simulink library "IO"  (R2024a)
settings: Solver=VariableStepAuto  StartTime=0.0  StopTime=10.0  RelTol=1e-3
values from neighbouring files (symbols this model uses):
  ADCBits = 12.0    [IO.sldd]
  DigitalPolarity : value not decoded    [IO.sldd]
  Vref = 5.0    [IO.sldd]
undefined symbols (not defined in the file or in its folder): Bridge, dt, enum2Raptor, H, raptor_xcp_function
libraries: Raptor_lib x118, Utilities x27, Cooling x1
(part 4 of 4)

== system IO/CANOutputs/Brake ==
  IO_CAN2_151_Bus : Inport
  Bus Selector : BusSelector  OutputSignals=IO_BrakeBias_pct,IO_BrakePressureF_psi,IO_BrakePressureR_psi
  RollingCounterGenerator : Utilities/RollingCounterGenerator
  raptor_can_txmsg : Raptor_lib/CAN/raptor_can_txmsg  canDefinition=struct('dbcFile', 'raptor_CAN2.dbc','message', 'VCU_151','comment', '','signals', {{'VCU_brakeBias','VCU_brakePressureF','VCU_brakePressureR','VCU_counterMsg151'}},'enabled', [ 1 1 1 1;],'scaled', [ 1 1 1 1;],'canBus', '''CAN2''','messageID', [ 151;],'idMask', [ 536870911;],'payloadMask', [],'payloadValue', [],'useDbcPeriod', [ 0;],'period', [ 100;],'queueSize', [ 1;],'label', [ 0;],'ver', [ 2;],'showID', [ 0;],'showRaw', [ 0;],'showRawMsg', [ 0;],'useStartVals', [ 0;],'extendedId', [ 0;],'useSimFunc', [ 0;],'sim_func_name', '''''','fill', [ 0;],'editID', [ 0;],'signalOrder', [ 1;],'signalAscDes', [ 1;],'msgLength', [ 8;])  canBus='CAN2'  queueSize=1  payloadMask=[]  payloadValue=[]  period=100  showID=0  label=0  idMask=hex2dec('1FFFFFFF')  fill=0  id=151  showRaw=0  signalOrder=1  signalInfo={{struct('Name', 'VCU_brakePressureR','StartBit', [ 48;],'SignalSize', [ 16;],'ByteOrder', 'LittleEndian','ValueType', 'SIGNED','Class', 'int16','Signed', [ 1;],'Factor', [ 0.1;],'Offset', [ 0;],'Min', [ 0;],'Max', [ 2000;],'Units', 'psi','StartVal', [ 0;],'Comment', 'Rear brake pressure sensor','Multiplexed', [ 0;],'Multiplexor', [ 0;],'MultiplexMode_Min', [],'MultiplexMode_Max', []),struct('Name', 'VCU_brakePressureF','StartBit', [ 32;],'SignalSize', [ 16;],'ByteOrder', 'LittleEndian','ValueType', 'SIGNED','Class', 'int16','Signed', [ 1;],'Factor', [ 0.1;],'Offset', [ 0;],'Min', [ 0;],'Max', [ 2000;],'Units', 'psi','StartVal', [ 0;],'Comment', 'Front brake pressure sensor','Multiplexed', [ 0;],'Multiplexor', [ 0;],'MultiplexMode_Min', [],'MultiplexMode_Max', []),struct('Name', 'VCU_brakeBias','StartBit', [ 16;],'SignalSize', [ 16;],'ByteOrder', 'LittleEndian','ValueType', 'SIGNED','Class', 'int16','Signed', [ 1;],'Factor', [ 0.1;],'Offset', [ 0;],'Min', [ -3276.8;],'Max', [ 3276.7;],'Units', '%','StartVal', [ 0;],'Comment', 'Brake bias','Multiplexed', [ 0;],'Multiplexor', [ 0;],'MultiplexMode_Min', [],'MultiplexMode_Max', []),struct('Name', 'VCU_counterMsg151','StartBit', [ 0;],'SignalSize', [ 4;],'ByteOrder', 'LittleEndian','ValueType', 'UNSIGNED','Class', 'uint8','Signed', [ 0;],'Factor', [ 1;],'Offset', [ 0;],'Min', [ 0;],'Max', [ 15;],'Units', '','StartVal', [ 0;],'Comment', 'Counter Message 151','Multiplexed', [ 0;],'Multiplexor', [ 0;],'MultiplexMode_Min', [],'MultiplexMode_Max', [])}}  useSimFunc=0  sim_func_name=''  useStartVals=0
      settings: SourceProductName=Raptor
  raptor_function_call_collector : Raptor_lib/Triggers/raptor_function_call_collector  count=10
      settings: SourceProductName=Raptor
  wires:
  raptor_function_call_collector/1 -> RollingCounterGenerator/Trigger
  RollingCounterGenerator/1 -> raptor_can_txmsg/4
  Bus Selector/3 -> raptor_can_txmsg/3  "<IO_BrakePressureR_psi>"
  Bus Selector/1 -> raptor_can_txmsg/1  "<IO_BrakeBias_pct>"
  Bus Selector/2 -> raptor_can_txmsg/2  "<IO_BrakePressureF_psi>"
  IO_CAN2_151_Bus/1 -> Bus Selector/1

== system IO/CANOutputs/DCDC ==
  IO_CAN1_18008FD0_Bus : Inport
  Bus Selector : BusSelector  OutputSignals=IO_DCDCEnable_bool
  Ground : Ground
  raptor_can_txmsg : Raptor_lib/CAN/raptor_can_txmsg  canDefinition=struct('dbcFile', 'raptor_CAN1.dbc','message', 'VCU_18008FD0','comment', '','signals', {{'VCU_dcdcEnable','VCU_dcdcProtect'}},'enabled', [ 1 1;],'scaled', [ 1 1;],'canBus', '''CAN1''','messageID', [ 402690000;],'idMask', [ 536870911;],'payloadMask', [],'payloadValue', [],'useDbcPeriod', [ 0;],'period', [ 100;],'queueSize', [ 1;],'label', [ 0;],'ver', [ 2;],'showID', [ 0;],'showRaw', [ 0;],'showRawMsg', [ 0;],'useStartVals', [ 0;],'extendedId', [ 1;],'useSimFunc', [ 0;],'sim_func_name', '''''','fill', [ 0;],'editID', [ 0;],'signalOrder', [ 1;],'signalAscDes', [ 1;],'msgLength', [ 8;])  canBus='CAN1'  queueSize=1  payloadMask=[]  payloadValue=[]  period=100  showID=0  label=0  idMask=hex2dec('1FFFFFFF')  fill=0  id=402690000  showRaw=0  signalOrder=1  signalInfo={{struct('Name', 'VCU_dcdcProtect','StartBit', [ 2;],'SignalSize', [ 2;],'ByteOrder', 'BigEndian','ValueType', 'UNSIGNED','Class', 'uint8','Signed', [ 0;],'Factor', [ 1;],'Offset', [ 0;],'Min', [ 0;],'Max', [ 0;],'Units', '','StartVal', [ 0;],'Comment', 'Protect command - once commanded, converter won`t work until restart (decimal); 1: protection confirmed','Multiplexed', [ 0;],'Multiplexor', [ 0;],'MultiplexMode_Min', [],'MultiplexMode_Max', []),struct('Name', 'VCU_dcdcEnable','StartBit', [ 0;],'SignalSize', [ 2;],'ByteOrder', 'BigEndian','ValueType', 'UNSIGNED','Class', 'uint8','Signed', [ 0;],'Factor', [ 1;],'Offset', [ 0;],'Min', [ 0;],'Max', [ 0;],'Units', '','StartVal', [ 0;],'Comment', 'Enable command (decimal); 1: enable, 2: disable','Multiplexed', [ 0;],'Multiplexor', [ 0;],'MultiplexMode_Min', [],'MultiplexMode_Max', [])}}  useSimFunc=0  sim_func_name=''  useStartVals=0
      settings: SourceProductName=Raptor
  wires:
  Ground/1 -> raptor_can_txmsg/2
  Bus Selector/1 -> raptor_can_txmsg/1  "<IO_DCDCEnable_bool>"
  IO_CAN1_18008FD0_Bus/1 -> Bus Selector/1

== system IO/CANOutputs/Front Left Tire Temp ==
  IO_CAN2_156_Bus : Inport
  Bus Selector : BusSelector  OutputSignals=IN_TireTempFLI_degC,IN_TireTempFLM_degC,IN_TireTempFLO_degC
  RollingCounterGenerator : Utilities/RollingCounterGenerator
  raptor_can_txmsg : Raptor_lib/CAN/raptor_can_txmsg  canDefinition=struct('dbcFile', 'raptor_CAN2.dbc','message', 'VCU_156','comment', '','signals', {{'VCU_counterMsg156','VCU_tireTempFLI','VCU_tireTempFLM','VCU_tireTempFLO'}},'enabled', [ 1 1 1 1;],'scaled', [ 1 1 1 1;],'canBus', '''CAN2''','messageID', [ 156;],'idMask', [ 536870911;],'payloadMask', [],'payloadValue', [],'useDbcPeriod', [ 0;],'period', [ 100;],'queueSize', [ 1;],'label', [ 0;],'ver', [ 2;],'showID', [ 0;],'showRaw', [ 0;],'showRawMsg', [ 0;],'useStartVals', [ 0;],'extendedId', [ 0;],'useSimFunc', [ 0;],'sim_func_name', '''''','fill', [ 0;],'editID', [ 0;],'signalOrder', [ 1;],'signalAscDes', [ 1;],'msgLength', [ 8;])  canBus='CAN2'  queueSize=1  payloadMask=[]  payloadValue=[]  period=100  showID=0  label=0  idMask=hex2dec('1FFFFFFF')  fill=0  id=156  showRaw=0  signalOrder=1  signalInfo={{struct('Name', 'VCU_counterMsg156','StartBit', [ 0;],'SignalSize', [ 4;],'ByteOrder', 'LittleEndian','ValueType', 'UNSIGNED','Class', 'uint8','Signed', [ 0;],'Factor', [ 1;],'Offset', [ 0;],'Min', [ 0;],'Max', [ 15;],'Units', '','StartVal', [ 0;],'Comment', 'Counter Message 156','Multiplexed', [ 0;],'Multiplexor', [ 0;],'MultiplexMode_Min', [],'MultiplexMode_Max', []),struct('Name', 'VCU_tireTempFLI','StartBit', [ 16;],'SignalSize', [ 16;],'ByteOrder', 'LittleEndian','ValueType', 'SIGNED','Class', 'int16','Signed', [ 1;],'Factor', [ 0.1;],'Offset', [ 0;],'Min', [ -3276.8;],'Max', [ 3276.7;],'Units', 'degC','StartVal', [ 0;],'Comment', 'FLI tire temperature','Multiplexed', [ 0;],'Multiplexor', [ 0;],'MultiplexMode_Min', [],'MultiplexMode_Max', []),struct('Name', 'VCU_tireTempFLM','StartBit', [ 32;],'SignalSize', [ 16;],'ByteOrder', 'LittleEndian','ValueType', 'SIGNED','Class', 'int16','Signed', [ 1;],'Factor', [ 0.1;],'Offset', [ 0;],'Min', [ -3276.8;],'Max', [ 3276.7;],'Units', 'degC','StartVal', [ 0;],'Comment', 'FLM tire temperature','Multiplexed', [ 0;],'Multiplexor', [ 0;],'MultiplexMode_Min', [],'MultiplexMode_Max', []),struct('Name', 'VCU_tireTempFLO','StartBit', [ 48;],'SignalSize', [ 16;],'ByteOrder', 'LittleEndian','ValueType', 'SIGNED','Class', 'int16','Signed', [ 1;],'Factor', [ 0.1;],'Offset', [ 0;],'Min', [ -3276.8;],'Max', [ 3276.7;],'Units', 'degC','StartVal', [ 0;],'Comment', 'FLO tire temperature','Multiplexed', [ 0;],'Multiplexor', [ 0;],'MultiplexMode_Min', [],'MultiplexMode_Max', [])}}  useSimFunc=0  sim_func_name=''  useStartVals=0
      settings: SourceProductName=Raptor
  raptor_function_call_collector : Raptor_lib/Triggers/raptor_function_call_collector  count=10
      settings: SourceProductName=Raptor
  wires:
  raptor_function_call_collector/1 -> RollingCounterGenerator/Trigger
  RollingCounterGenerator/1 -> raptor_can_txmsg/1
  Bus Selector/3 -> raptor_can_txmsg/4  "<IN_TireTempFLO_degC>"
  Bus Selector/2 -> raptor_can_txmsg/3  "<IN_TireTempFLM_degC>"
  Bus Selector/1 -> raptor_can_txmsg/2  "<IN_TireTempFLI_degC>"
  IO_CAN2_156_Bus/1 -> Bus Selector/1

== system IO/CANOutputs/Front Right Tire Temp ==
  IO_CAN2_157_Bus : Inport
  Bus Selector : BusSelector  OutputSignals=IN_TireTempFRI_degC,IN_TireTempFRM_degC,IN_TireTempFRO_degC
  RollingCounterGenerator : Utilities/RollingCounterGenerator
  raptor_can_txmsg : Raptor_lib/CAN/raptor_can_txmsg  canDefinition=struct('dbcFile', 'raptor_CAN2.dbc','message', 'VCU_157','comment', '','signals', {{'VCU_counterMsg157','VCU_tireTempFRI','VCU_tireTempFRM','VCU_tireTempFRO'}},'enabled', [ 1 1 1 1;],'scaled', [ 1 1 1 1;],'canBus', '''CAN2''','messageID', [ 157;],'idMask', [ 536870911;],'payloadMask', [],'payloadValue', [],'useDbcPeriod', [ 0;],'period', [ 100;],'queueSize', [ 1;],'label', [ 0;],'ver', [ 2;],'showID', [ 0;],'showRaw', [ 0;],'showRawMsg', [ 0;],'useStartVals', [ 0;],'extendedId', [ 0;],'useSimFunc', [ 0;],'sim_func_name', '''''','fill', [ 0;],'editID', [ 0;],'signalOrder', [ 1;],'signalAscDes', [ 1;],'msgLength', [ 8;])  canBus='CAN2'  queueSize=1  payloadMask=[]  payloadValue=[]  period=100  showID=0  label=0  idMask=hex2dec('1FFFFFFF')  fill=0  id=157  showRaw=0  signalOrder=1  signalInfo={{struct('Name', 'VCU_counterMsg157','StartBit', [ 0;],'SignalSize', [ 4;],'ByteOrder', 'LittleEndian','ValueType', 'UNSIGNED','Class', 'uint8','Signed', [ 0;],'Factor', [ 1;],'Offset', [ 0;],'Min', [ 0;],'Max', [ 15;],'Units', '','StartVal', [ 0;],'Comment', 'Counter Message 157','Multiplexed', [ 0;],'Multiplexor', [ 0;],'MultiplexMode_Min', [],'MultiplexMode_Max', []),struct('Name', 'VCU_tireTempFRI','StartBit', [ 16;],'SignalSize', [ 16;],'ByteOrder', 'LittleEndian','ValueType', 'SIGNED','Class', 'int16','Signed', [ 1;],'Factor', [ 0.1;],'Offset', [ 0;],'Min', [ -3276.8;],'Max', [ 3276.7;],'Units', 'degC','StartVal', [ 0;],'Comment', 'FRI tire temperature','Multiplexed', [ 0;],'Multiplexor', [ 0;],'MultiplexMode_Min', [],'MultiplexMode_Max', []),struct('Name', 'VCU_tireTempFRM','StartBit', [ 32;],'SignalSize', [ 16;],'ByteOrder', 'LittleEndian','ValueType', 'SIGNED','Class', 'int16','Signed', [ 1;],'Factor', [ 0.1;],'Offset', [ 0;],'Min', [ -3276.8;],'Max', [ 3276.7;],'Units', 'degC','StartVal', [ 0;],'Comment', 'FRM tire temperature','Multiplexed', [ 0;],'Multiplexor', [ 0;],'MultiplexMode_Min', [],'MultiplexMode_Max', []),struct('Name', 'VCU_tireTempFRO','StartBit', [ 48;],'SignalSize', [ 16;],'ByteOrder', 'LittleEndian','ValueType', 'SIGNED','Class', 'int16','Signed', [ 1;],'Factor', [ 0.1;],'Offset', [ 0;],'Min', [ -3276.8;],'Max', [ 3276.7;],'Units', 'degC','StartVal', [ 0;],'Comment', 'FRO tire temperature','Multiplexed', [ 0;],'Multiplexor', [ 0;],'MultiplexMode_Min', [],'MultiplexMode_Max', [])}}  useSimFunc=0  sim_func_name=''  useStartVals=0
      settings: SourceProductName=Raptor
  raptor_function_call_collector : Raptor_lib/Triggers/raptor_function_call_collector  count=10
      settings: SourceProductName=Raptor
  wires:
  raptor_function_call_collector/1 -> RollingCounterGenerator/Trigger
  RollingCounterGenerator/1 -> raptor_can_txmsg/1
  Bus Selector/3 -> raptor_can_txmsg/4  "<IN_TireTempFRO_degC>"
  Bus Selector/2 -> raptor_can_txmsg/3  "<IN_TireTempFRM_degC>"
  Bus Selector/1 -> raptor_can_txmsg/2  "<IN_TireTempFRI_degC>"
  IO_CAN2_157_Bus/1 -> Bus Selector/1

== system IO/CANOutputs/Front Rotor Temp ==
  IO_CAN2_154_Bus : Inport
  Bus Selector : BusSelector  OutputSignals=IN_RotorTempFL_degC,IN_RotorTempFR_degC
  RollingCounterGenerator : Utilities/RollingCounterGenerator
  raptor_can_txmsg : Raptor_lib/CAN/raptor_can_txmsg  canDefinition=struct('dbcFile', 'raptor_CAN2.dbc','message', 'VCU_154','comment', '','signals', {{'VCU_counterMsg154','VCU_rotorTempFL','VCU_rotorTempFR'}},'enabled', [ 1 1 1;],'scaled', [ 1 1 1;],'canBus', '''CAN2''','messageID', [ 154;],'idMask', [ 536870911;],'payloadMask', [],'payloadValue', [],'useDbcPeriod', [ 0;],'period', [ 100;],'queueSize', [ 1;],'label', [ 0;],'ver', [ 2;],'showID', [ 0;],'showRaw', [ 0;],'showRawMsg', [ 0;],'useStartVals', [ 0;],'extendedId', [ 0;],'useSimFunc', [ 0;],'sim_func_name', '''''','fill', [ 0;],'editID', [ 0;],'signalOrder', [ 1;],'signalAscDes', [ 1;],'msgLength', [ 8;])  canBus='CAN2'  queueSize=1  payloadMask=[]  payloadValue=[]  period=100  showID=0  label=0  idMask=hex2dec('1FFFFFFF')  fill=0  id=154  showRaw=0  signalOrder=1  signalInfo={{struct('Name', 'VCU_counterMsg154','StartBit', [ 0;],'SignalSize', [ 4;],'ByteOrder', 'LittleEndian','ValueType', 'UNSIGNED','Class', 'uint8','Signed', [ 0;],'Factor', [ 1;],'Offset', [ 0;],'Min', [ 0;],'Max', [ 15;],'Units', '','StartVal', [ 0;],'Comment', 'Counter Message 154','Multiplexed', [ 0;],'Multiplexor', [ 0;],'MultiplexMode_Min', [],'MultiplexMode_Max', []),struct('Name', 'VCU_rotorTempFL','StartBit', [ 16;],'SignalSize', [ 16;],'ByteOrder', 'LittleEndian','ValueType', 'SIGNED','Class', 'int16','Signed', [ 1;],'Factor', [ 0.1;],'Offset', [ 0;],'Min', [ -3276.8;],'Max', [ 3276.7;],'Units', 'degC','StartVal', [ 0;],'Comment', 'FL rotor temperature','Multiplexed', [ 0;],'Multiplexor', [ 0;],'MultiplexMode_Min', [],'MultiplexMode_Max', []),struct('Name', 'VCU_rotorTempFR','StartBit', [ 32;],'SignalSize', [ 16;],'ByteOrder', 'LittleEndian','ValueType', 'SIGNED','Class', 'int16','Signed', [ 1;],'Factor', [ 0.1;],'Offset', [ 0;],'Min', [ -3276.8;],'Max', [ 3276.7;],'Units', 'degC','StartVal', [ 0;],'Comment', '','Multiplexed', [ 0;],'Multiplexor', [ 0;],'MultiplexMode_Min', [],'MultiplexMode_Max', [])}}  useSimFunc=0  sim_func_name=''  useStartVals=0
      settings: SourceProductName=Raptor
  raptor_function_call_collector : Raptor_lib/Triggers/raptor_function_call_collector  count=10
      settings: SourceProductName=Raptor
  wires:
  RollingCounterGenerator/1 -> raptor_can_txmsg/1
  raptor_function_call_collector/1 -> RollingCounterGenerator/Trigger
  Bus Selector/2 -> raptor_can_txmsg/3  "<IN_RotorTempFR_degC>"
  Bus Selector/1 -> raptor_can_txmsg/2  "<IN_RotorTempFL_degC>"
  IO_CAN2_154_Bus/1 -> Bus Selector/1

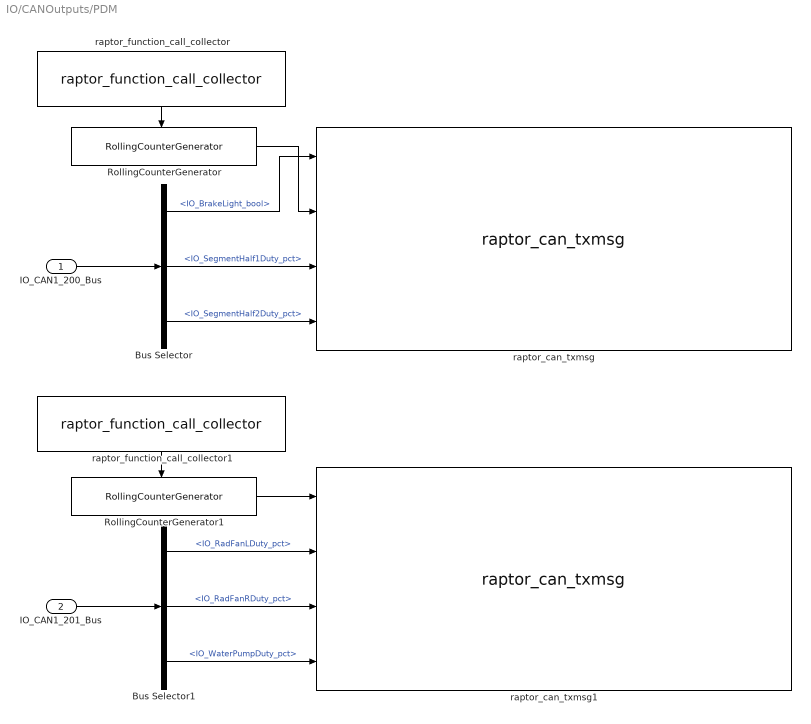
== system IO/CANOutputs/PDM ==
  IO_CAN1_200_Bus : Inport
  IO_CAN1_201_Bus : Inport  Port=2
  Bus Selector : BusSelector  OutputSignals=IO_BrakeLight_bool,IO_SegmentHalf1Duty_pct,IO_SegmentHalf2Duty_pct
  Bus Selector1 : BusSelector  OutputSignals=IO_RadFanLDuty_pct,IO_RadFanRDuty_pct,IO_WaterPumpDuty_pct
  RollingCounterGenerator : Utilities/RollingCounterGenerator
  RollingCounterGenerator1 : Utilities/RollingCounterGenerator
  raptor_can_txmsg : Raptor_lib/CAN/raptor_can_txmsg  canDefinition=struct('dbcFile', 'raptor_CAN1.dbc','message', 'VCU_200','comment', '','signals', {{'VCU_brakeLightCmd','VCU_counterMsg200','VCU_segmentHalf1Duty','VCU_segmentHalf2Duty'}},'enabled', [ 1 1 1 1;],'scaled', [ 1 1 1 1;],'canBus', '''CAN1''','messageID', [ 200;],'idMask', [ 536870911;],'payloadMask', [],'payloadValue', [],'useDbcPeriod', [ 0;],'period', [ 100;],'queueSize', [ 1;],'label', [ 0;],'ver', [ 2;],'showID', [ 0;],'showRaw', [ 0;],'showRawMsg', [ 0;],'useStartVals', [ 0;],'extendedId', [ 0;],'useSimFunc', [ 0;],'sim_func_name', '''''','fill', [ 0;],'editID', [ 0;],'signalOrder', [ 1;],'signalAscDes', [ 1;],'msgLength', [ 8;])  canBus='CAN1'  queueSize=1  payloadMask=[]  payloadValue=[]  period=100  showID=0  label=0  idMask=hex2dec('1FFFFFFF')  fill=0  id=200  showRaw=0  signalOrder=1  signalInfo={{struct('Name', 'VCU_segmentHalf2Duty','StartBit', [ 32;],'SignalSize', [ 16;],'ByteOrder', 'LittleEndian','ValueType', 'SIGNED','Class', 'int16','Signed', [ 1;],'Factor', [ 0.1;],'Offset', [ 0;],'Min', [ 0;],'Max', [ 100;],'Units', '%','StartVal', [ 0;],'Comment', 'Segment half 2 duty','Multiplexed', [ 0;],'Multiplexor', [ 0;],'MultiplexMode_Min', [],'MultiplexMode_Max', []),struct('Name', 'VCU_segmentHalf1Duty','StartBit', [ 16;],'SignalSize', [ 16;],'ByteOrder', 'LittleEndian','ValueType', 'SIGNED','Class', 'int16','Signed', [ 1;],'Factor', [ 0.1;],'Offset', [ 0;],'Min', [ 0;],'Max', [ 100;],'Units', '%','StartVal', [ 0;],'Comment', 'Segment half 1 duty','Multiplexed', [ 0;],'Multiplexor', [ 0;],'MultiplexMode_Min', [],'MultiplexMode_Max', []),struct('Name', 'VCU_brakeLightCmd','StartBit', [ 8;],'SignalSize', [ 1;],'ByteOrder', 'LittleEndian','ValueType', 'UNSIGNED','Class', 'uint8','Signed', [ 0;],'Factor', [ 1;],'Offset', [ 0;],'Min', [ 0;],'Max', [ 1;],'Units', '','StartVal', [ 0;],'Comment', 'Brake light command','Multiplexed', [ 0;],'Multiplexor', [ 0;],'MultiplexMode_Min', [],'MultiplexMode_Max', []),struct('Name', 'VCU_counterMsg200','StartBit', [ 0;],'SignalSize', [ 4;],'ByteOrder', 'LittleEndian','ValueType', 'UNSIGNED','Class', 'uint8','Signed', [ 0;],'Factor', [ 1;],'Offset', [ 0;],'Min', [ 0;],'Max', [ 15;],'Units', '','StartVal', [ 0;],'Comment', 'Counter Message 200','Multiplexed', [ 0;],'Multiplexor', [ 0;],'MultiplexMode_Min', [],'MultiplexMode_Max', [])}}  useSimFunc=0  sim_func_name=''  useStartVals=0
      settings: SourceProductName=Raptor
  raptor_can_txmsg1 : Raptor_lib/CAN/raptor_can_txmsg  canDefinition=struct('dbcFile', 'raptor_CAN1.dbc','message', 'VCU_201','comment', '','signals', {{'VCU_counterMsg201','VCU_radFanLDuty','VCU_radFanRDuty','VCU_waterPumpDuty'}},'enabled', [ 1 1 1 1;],'scaled', [ 1 1 1 1;],'canBus', '''CAN1''','messageID', [ 201;],'idMask', [ 536870911;],'payloadMask', [],'payloadValue', [],'useDbcPeriod', [ 0;],'period', [ 100;],'queueSize', [ 1;],'label', [ 0;],'ver', [ 2;],'showID', [ 0;],'showRaw', [ 0;],'showRawMsg', [ 0;],'useStartVals', [ 0;],'extendedId', [ 0;],'useSimFunc', [ 0;],'sim_func_name', '''''','fill', [ 0;],'editID', [ 0;],'signalOrder', [ 1;],'signalAscDes', [ 1;],'msgLength', [ 8;])  canBus='CAN1'  queueSize=1  payloadMask=[]  payloadValue=[]  period=100  showID=0  label=0  idMask=hex2dec('1FFFFFFF')  fill=0  id=201  showRaw=0  signalOrder=1  signalInfo={{struct('Name', 'VCU_waterPumpDuty','StartBit', [ 48;],'SignalSize', [ 16;],'ByteOrder', 'LittleEndian','ValueType', 'SIGNED','Class', 'int16','Signed', [ 1;],'Factor', [ 0.1;],'Offset', [ 0;],'Min', [ 0;],'Max', [ 100;],'Units', '%','StartVal', [ 0;],'Comment', 'Water pump duty','Multiplexed', [ 0;],'Multiplexor', [ 0;],'MultiplexMode_Min', [],'MultiplexMode_Max', []),struct('Name', 'VCU_radFanRDuty','StartBit', [ 32;],'SignalSize', [ 16;],'ByteOrder', 'LittleEndian','ValueType', 'SIGNED','Class', 'int16','Signed', [ 1;],'Factor', [ 0.1;],'Offset', [ 0;],'Min', [ 0;],'Max', [ 100;],'Units', '%','StartVal', [ 0;],'Comment', 'Right radiator fan duty','Multiplexed', [ 0;],'Multiplexor', [ 0;],'MultiplexMode_Min', [],'MultiplexMode_Max', []),struct('Name', 'VCU_radFanLDuty','StartBit', [ 16;],'SignalSize', [ 16;],'ByteOrder', 'LittleEndian','ValueType', 'SIGNED','Class', 'int16','Signed', [ 1;],'Factor', [ 0.1;],'Offset', [ 0;],'Min', [ 0;],'Max', [ 100;],'Units', '%','StartVal', [ 0;],'Comment', 'Left radiator fan duty','Multiplexed', [ 0;],'Multiplexor', [ 0;],'MultiplexMode_Min', [],'MultiplexMode_Max', []),struct('Name', 'VCU_counterMsg201','StartBit', [ 0;],'SignalSize', [ 4;],'ByteOrder', 'LittleEndian','ValueType', 'UNSIGNED','Class', 'uint8','Signed', [ 0;],'Factor', [ 1;],'Offset', [ 0;],'Min', [ 0;],'Max', [ 15;],'Units', '','StartVal', [ 0;],'Comment', 'Counter Message 201','Multiplexed', [ 0;],'Multiplexor', [ 0;],'MultiplexMode_Min', [],'MultiplexMode_Max', [])}}  useSimFunc=0  sim_func_name=''  useStartVals=0
      settings: SourceProductName=Raptor
  raptor_function_call_collector : Raptor_lib/Triggers/raptor_function_call_collector  count=10
      settings: SourceProductName=Raptor
  raptor_function_call_collector1 : Raptor_lib/Triggers/raptor_function_call_collector  count=10
      settings: SourceProductName=Raptor
  wires:
  raptor_function_call_collector1/1 -> RollingCounterGenerator1/Trigger
  RollingCounterGenerator1/1 -> raptor_can_txmsg1/1
  Bus Selector1/1 -> raptor_can_txmsg1/2  "<IO_RadFanLDuty_pct>"
  Bus Selector1/3 -> raptor_can_txmsg1/4  "<IO_WaterPumpDuty_pct>"
  Bus Selector1/2 -> raptor_can_txmsg1/3  "<IO_RadFanRDuty_pct>"
  IO_CAN1_201_Bus/1 -> Bus Selector1/1
  raptor_function_call_collector/1 -> RollingCounterGenerator/Trigger
  RollingCounterGenerator/1 -> raptor_can_txmsg/2
  Bus Selector/1 -> raptor_can_txmsg/1  "<IO_BrakeLight_bool>"
  Bus Selector/3 -> raptor_can_txmsg/4  "<IO_SegmentHalf2Duty_pct>"
  Bus Selector/2 -> raptor_can_txmsg/3  "<IO_SegmentHalf1Duty_pct>"
  IO_CAN1_200_Bus/1 -> Bus Selector/1

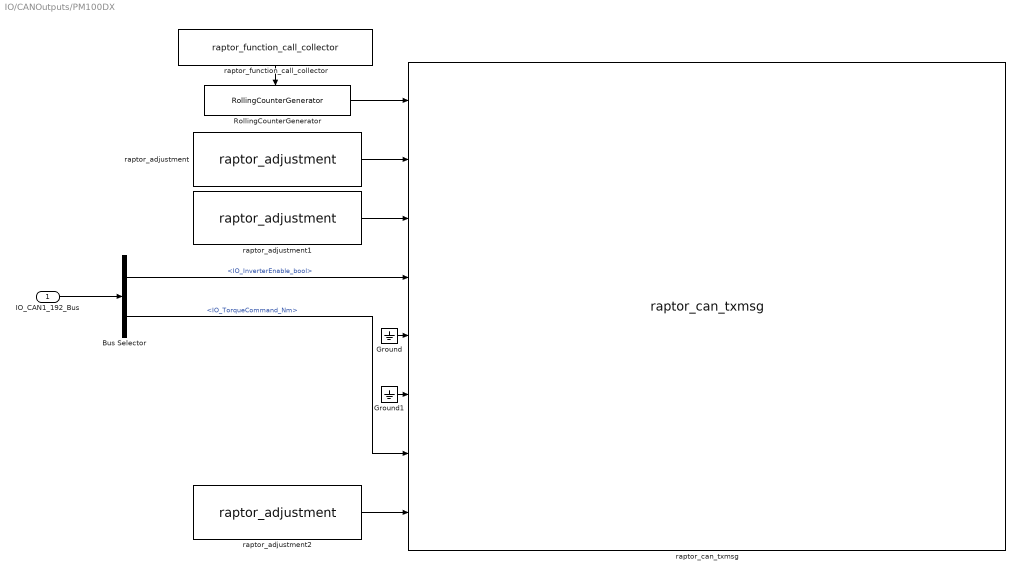
== system IO/CANOutputs/PM100DX ==
  IO_CAN1_192_Bus : Inport
  Bus Selector : BusSelector  OutputSignals=IO_InverterEnable_bool,IO_TorqueCommand_Nm
  Ground : Ground
  Ground1 : Ground
  RollingCounterGenerator : Utilities/RollingCounterGenerator
  raptor_adjustment : Raptor_lib/Data Storage/raptor_adjustment  paramName='IO_InverterDirectionCmd_bool'  nameSource=Parameter  initValue=1  dataType=boolean  storage=Calibration  calDispType=Number  calEnum={'False', 'True'}  calGain=1.0  calOffset=0.0  calMax=inf  calMin=-inf  calFormat='-1'  calUnit=''  calHelp=''  calAccess=1  calFunction=raptor_xcp_function(gcb)  calDispHeaders=off  calColHeaders={'Col1' 'Col2' 'Col3'}  calRowHeaders={'Row1' 'Row2' 'Row3'}
      settings: SourceProductName=Raptor
  raptor_adjustment1 : Raptor_lib/Data Storage/raptor_adjustment  paramName='IO_InverterDischargeCmd_bool'  nameSource=Parameter  initValue=0  dataType=boolean  storage=Calibration  calDispType=Number  calEnum={'False', 'True'}  calGain=1.0  calOffset=0.0  calMax=inf  calMin=-inf  calFormat='-1'  calUnit=''  calHelp=''  calAccess=1  calFunction=raptor_xcp_function(gcb)  calDispHeaders=off  calColHeaders={'Col1' 'Col2' 'Col3'}  calRowHeaders={'Row1' 'Row2' 'Row3'}
      settings: SourceProductName=Raptor
  raptor_adjustment2 : Raptor_lib/Data Storage/raptor_adjustment  paramName='IO_InverterTorqueLimit_Nm'  nameSource=Parameter  initValue=240  dataType=single  storage=Calibration  calDispType=Number  calEnum={'False', 'True'}  calGain=1.0  calOffset=0.0  calMax=inf  calMin=-inf  calFormat='-1'  calUnit=''  calHelp=''  calAccess=1  calFunction=raptor_xcp_function(gcb)  calDispHeaders=off  calColHeaders={'Col1' 'Col2' 'Col3'}  calRowHeaders={'Row1' 'Row2' 'Row3'}
      settings: SourceProductName=Raptor
  raptor_can_txmsg : Raptor_lib/CAN/raptor_can_txmsg  canDefinition=struct('dbcFile', 'raptor_CAN1.dbc','message', 'VCU_192','comment', '','signals', {{'VCU_counterMsg192','VCU_directionCommand','VCU_inverterDischarge','VCU_inverterEnable','VCU_speedCommand','VCU_speedModeEnable','VCU_torqueCommand','VCU_torqueLimitCommand'}},'enabled', [ 1 1 1 1 1 1 1 1;],'scaled', [ 1 1 1 1 1 1 1 1;],'canBus', '''CAN1''','messageID', [ 192;],'idMask', [ 536870911;],'payloadMask', [],'payloadValue', [],'useDbcPeriod', [ 0;],'period', [ 100;],'queueSize', [ 1;],'label', [ 0;],'ver', [ 2;],'showID', [ 0;],'showRaw', [ 0;],'showRawMsg', [ 0;],'useStartVals', [ 0;],'extendedId', [ 0;],'useSimFunc', [ 0;],'sim_func_name', '''''','fill', [ 0;],'editID', [ 0;],'signalOrder', [ 1;],'signalAscDes', [ 1;],'msgLength', [ 8;])  canBus='CAN1'  queueSize=1  payloadMask=[]  payloadValue=[]  period=100  showID=0  label=0  idMask=hex2dec('1FFFFFFF')  fill=0  id=192  showRaw=0  signalOrder=1  signalInfo={{struct('Name', 'VCU_torqueLimitCommand','StartBit', [ 48;],'SignalSize', [ 16;],'ByteOrder', 'LittleEndian','ValueType', 'SIGNED','Class', 'int16','Signed', [ 1;],'Factor', [ 0.1;],'Offset', [ 0;],'Min', [ -3276.8;],'Max', [ 3276.7;],'Units', 'Nm','StartVal', [ 0;],'Comment', 'Torque Limit - set to 0 to keep default','Multiplexed', [ 0;],'Multiplexor', [ 0;],'MultiplexMode_Min', [],'MultiplexMode_Max', []),struct('Name', 'VCU_torqueCommand','StartBit', [ 0;],'SignalSize', [ 16;],'ByteOrder', 'LittleEndian','ValueType', 'SIGNED','Class', 'int16','Signed', [ 1;],'Factor', [ 0.1;],'Offset', [ 0;],'Min', [ -3276.8;],'Max', [ 3276.7;],'Units', 'Nm','StartVal', [ 0;],'Comment', 'Torque Command in Torque Mode','Multiplexed', [ 0;],'Multiplexor', [ 0;],'MultiplexMode_Min', [],'MultiplexMode_Max', []),struct('Name', 'VCU_speedModeEnable','StartBit', [ 42;],'SignalSize', [ 1;],'ByteOrder', 'LittleEndian','ValueType', 'UNSIGNED','Class', 'uint8','Signed', [ 0;],'Factor', [ 1;],'Offset', [ 0;],'Min', [ 0;],'Max', [ 1;],'Units', '','StartVal', [ 0;],'Comment', '0 = No Change Mode, 1 = Change to Speed Mode from Torque Mode','Multiplexed', [ 0;],'Multiplexor', [ 0;],'MultiplexMode_Min', [],'MultiplexMode_Max', []),struct('Name', 'VCU_speedCommand','StartBit', [ 16;],'SignalSize', [ 16;],'ByteOrder', 'LittleEndian','ValueType', 'SIGNED','Class', 'int16','Signed', [ 1;],'Factor', [ 1;],'Offset', [ 0;],'Min', [ -32768;],'Max', [ 32767;],'Units', 'rpm','StartVal', [ 0;],'Comment', 'Speed Command when used in Speed Mode','Multiplexed', [ 0;],'Multiplexor', [ 0;],'MultiplexMode_Min', [],'MultiplexMode_Max', []),struct('Name', 'VCU_counterMsg192','StartBit', [ 44;],'SignalSize', [ 4;],'ByteOrder', 'LittleEndian','ValueType', 'UNSIGNED','Class', 'uint8','Signed', [ 0;],'Factor', [ 1;],'Offset', [ 0;],'Min', [ 0;],'Max', [ 15;],'Units', '','StartVal', [ 0;],'Comment', 'Counter Message 192','Multiplexed', [ 0;],'Multiplexor', [ 0;],'MultiplexMode_Min', [],'MultiplexMode_Max', []),struct('Name', 'VCU_inverterEnable','StartBit', [ 40;],'SignalSize', [ 1;],'ByteOrder', 'LittleEndian','ValueType', 'UNSIGNED','Class', 'uint8','Signed', [ 0;],'Factor', [ 1;],'Offset', [ 0;],'Min', [ 0;],'Max', [ 1;],'Units', '','StartVal', [ 0;],'Comment', '0 = Inverter OFF, 1 = Inverter ON','Multiplexed', [ 0;],'Multiplexor', [ 0;],'MultiplexMode_Min', [],'MultiplexMode_Max', []),struct('Name', 'VCU_inverterDischarge','StartBit', [ 41;],'SignalSize', [ 1;],'ByteOrder', 'LittleEndian','ValueType', 'UNSIGNED','Class', 'uint8','Signed', [ 0;],'Factor', [ 1;],'Offset', [ 0;],'Min', [ 0;],'Max', [ 1;],'Units', '','StartVal', [ 0;],'Comment', '0 = Discharge Disable, 1 = Discharge Enable','Multiplexed', [ 0;],'Multiplexor', [ 0;],'MultiplexMode_Min', [],'MultiplexMode_Max', []),struct('Name', 'VCU_directionCommand','StartBit', [ 32;],'SignalSize', [ 1;],'ByteOrder', 'LittleEndian','ValueType', 'UNSIGNED','Class', 'uint8','Signed', [ 0;],'Factor', [ 1;],'Offset', [ 0;],'Min', [ 0;],'Max', [ 1;],'Units', '','StartVal', [ 0;],'Comment', '0 = CW, 1 = CCW, viewed from the shaft end of the motor','Multiplexed', [ 0;],'Multiplexor', [ 0;],'MultiplexMode_Min', [],'MultiplexMode_Max', [])}}  useSimFunc=0  sim_func_name=''  useStartVals=0
      settings: SourceProductName=Raptor
  raptor_function_call_collector : Raptor_lib/Triggers/raptor_function_call_collector  count=10
      settings: SourceProductName=Raptor
  wires:
  raptor_function_call_collector/1 -> RollingCounterGenerator/Trigger
  raptor_adjustment2/1 -> raptor_can_txmsg/8
  raptor_adjustment1/1 -> raptor_can_txmsg/3
  raptor_adjustment/1 -> raptor_can_txmsg/2
  RollingCounterGenerator/1 -> raptor_can_txmsg/1
  Ground1/1 -> raptor_can_txmsg/6
  Ground/1 -> raptor_can_txmsg/5
  Bus Selector/2 -> raptor_can_txmsg/7  "<IO_TorqueCommand_Nm>"
  Bus Selector/1 -> raptor_can_txmsg/4  "<IO_InverterEnable_bool>"
  IO_CAN1_192_Bus/1 -> Bus Selector/1

== system IO/CANOutputs/Rear Left Tire Temp ==
  IO_CAN2_158_Bus : Inport
  Bus Selector : BusSelector  OutputSignals=IN_TireTempRLI_degC,IN_TireTempRLM_degC,IN_TireTempRLO_degC
  RollingCounterGenerator : Utilities/RollingCounterGenerator
  raptor_can_txmsg : Raptor_lib/CAN/raptor_can_txmsg  canDefinition=struct('dbcFile', 'raptor_CAN2.dbc','message', 'VCU_158','comment', '','signals', {{'VCU_counterMsg158','VCU_tireTempRLI','VCU_tireTempRLM','VCU_tireTempRLO'}},'enabled', [ 1 1 1 1;],'scaled', [ 1 1 1 1;],'canBus', '''CAN2''','messageID', [ 158;],'idMask', [ 536870911;],'payloadMask', [],'payloadValue', [],'useDbcPeriod', [ 0;],'period', [ 100;],'queueSize', [ 1;],'label', [ 0;],'ver', [ 2;],'showID', [ 0;],'showRaw', [ 0;],'showRawMsg', [ 0;],'useStartVals', [ 0;],'extendedId', [ 0;],'useSimFunc', [ 0;],'sim_func_name', '''''','fill', [ 0;],'editID', [ 0;],'signalOrder', [ 1;],'signalAscDes', [ 1;],'msgLength', [ 8;])  canBus='CAN2'  queueSize=1  payloadMask=[]  payloadValue=[]  period=100  showID=0  label=0  idMask=hex2dec('1FFFFFFF')  fill=0  id=158  showRaw=0  signalOrder=1  signalInfo={{struct('Name', 'VCU_counterMsg158','StartBit', [ 0;],'SignalSize', [ 4;],'ByteOrder', 'LittleEndian','ValueType', 'UNSIGNED','Class', 'uint8','Signed', [ 0;],'Factor', [ 1;],'Offset', [ 0;],'Min', [ 0;],'Max', [ 15;],'Units', '','StartVal', [ 0;],'Comment', 'Counter Message 158','Multiplexed', [ 0;],'Multiplexor', [ 0;],'MultiplexMode_Min', [],'MultiplexMode_Max', []),struct('Name', 'VCU_tireTempRLI','StartBit', [ 16;],'SignalSize', [ 16;],'ByteOrder', 'LittleEndian','ValueType', 'SIGNED','Class', 'int16','Signed', [ 1;],'Factor', [ 0.1;],'Offset', [ 0;],'Min', [ -3276.8;],'Max', [ 3276.7;],'Units', 'degC','StartVal', [ 0;],'Comment', 'RLI tire temperature','Multiplexed', [ 0;],'Multiplexor', [ 0;],'MultiplexMode_Min', [],'MultiplexMode_Max', []),struct('Name', 'VCU_tireTempRLM','StartBit', [ 32;],'SignalSize', [ 16;],'ByteOrder', 'LittleEndian','ValueType', 'SIGNED','Class', 'int16','Signed', [ 1;],'Factor', [ 0.1;],'Offset', [ 0;],'Min', [ -3276.8;],'Max', [ 3276.7;],'Units', 'degC','StartVal', [ 0;],'Comment', 'RLM tire temperature','Multiplexed', [ 0;],'Multiplexor', [ 0;],'MultiplexMode_Min', [],'MultiplexMode_Max', []),struct('Name', 'VCU_tireTempRLO','StartBit', [ 48;],'SignalSize', [ 16;],'ByteOrder', 'LittleEndian','ValueType', 'SIGNED','Class', 'int16','Signed', [ 1;],'Factor', [ 0.1;],'Offset', [ 0;],'Min', [ -3276.8;],'Max', [ 3276.7;],'Units', 'degC','StartVal', [ 0;],'Comment', 'RLO tire temperature','Multiplexed', [ 0;],'Multiplexor', [ 0;],'MultiplexMode_Min', [],'MultiplexMode_Max', [])}}  useSimFunc=0  sim_func_name=''  useStartVals=0
      settings: SourceProductName=Raptor
  raptor_function_call_collector : Raptor_lib/Triggers/raptor_function_call_collector  count=10
      settings: SourceProductName=Raptor
  wires:
  raptor_function_call_collector/1 -> RollingCounterGenerator/Trigger
  RollingCounterGenerator/1 -> raptor_can_txmsg/1
  Bus Selector/3 -> raptor_can_txmsg/4  "<IN_TireTempRLO_degC>"
  Bus Selector/2 -> raptor_can_txmsg/3  "<IN_TireTempRLM_degC>"
  Bus Selector/1 -> raptor_can_txmsg/2  "<IN_TireTempRLI_degC>"
  IO_CAN2_158_Bus/1 -> Bus Selector/1

== system IO/CANOutputs/Rear Right Tire Temp ==
  IO_CAN2_159_Bus : Inport
  Bus Selector : BusSelector  OutputSignals=IN_TireTempRRI_degC,IN_TireTempRRM_degC,IN_TireTempRRO_degC
  RollingCounterGenerator : Utilities/RollingCounterGenerator
  raptor_can_txmsg : Raptor_lib/CAN/raptor_can_txmsg  canDefinition=struct('dbcFile', 'raptor_CAN2.dbc','message', 'VCU_159','comment', '','signals', {{'VCU_counterMsg159','VCU_tireTempRRI','VCU_tireTempRRM','VCU_tireTempRRO'}},'enabled', [ 1 1 1 1;],'scaled', [ 1 1 1 1;],'canBus', '''CAN2''','messageID', [ 159;],'idMask', [ 536870911;],'payloadMask', [],'payloadValue', [],'useDbcPeriod', [ 0;],'period', [ 100;],'queueSize', [ 1;],'label', [ 0;],'ver', [ 2;],'showID', [ 0;],'showRaw', [ 0;],'showRawMsg', [ 0;],'useStartVals', [ 0;],'extendedId', [ 0;],'useSimFunc', [ 0;],'sim_func_name', '''''','fill', [ 0;],'editID', [ 0;],'signalOrder', [ 1;],'signalAscDes', [ 1;],'msgLength', [ 8;])  canBus='CAN2'  queueSize=1  payloadMask=[]  payloadValue=[]  period=100  showID=0  label=0  idMask=hex2dec('1FFFFFFF')  fill=0  id=159  showRaw=0  signalOrder=1  signalInfo={{struct('Name', 'VCU_counterMsg159','StartBit', [ 0;],'SignalSize', [ 4;],'ByteOrder', 'LittleEndian','ValueType', 'UNSIGNED','Class', 'uint8','Signed', [ 0;],'Factor', [ 1;],'Offset', [ 0;],'Min', [ 0;],'Max', [ 15;],'Units', '','StartVal', [ 0;],'Comment', 'Counter Message 159','Multiplexed', [ 0;],'Multiplexor', [ 0;],'MultiplexMode_Min', [],'MultiplexMode_Max', []),struct('Name', 'VCU_tireTempRRI','StartBit', [ 16;],'SignalSize', [ 16;],'ByteOrder', 'LittleEndian','ValueType', 'SIGNED','Class', 'int16','Signed', [ 1;],'Factor', [ 0.1;],'Offset', [ 0;],'Min', [ -3276.8;],'Max', [ 3276.7;],'Units', 'degC','StartVal', [ 0;],'Comment', 'RRI tire temperature','Multiplexed', [ 0;],'Multiplexor', [ 0;],'MultiplexMode_Min', [],'MultiplexMode_Max', []),struct('Name', 'VCU_tireTempRRM','StartBit', [ 32;],'SignalSize', [ 16;],'ByteOrder', 'LittleEndian','ValueType', 'SIGNED','Class', 'int16','Signed', [ 1;],'Factor', [ 0.1;],'Offset', [ 0;],'Min', [ -3276.8;],'Max', [ 3276.7;],'Units', 'degC','StartVal', [ 0;],'Comment', 'RRM tire temperature','Multiplexed', [ 0;],'Multiplexor', [ 0;],'MultiplexMode_Min', [],'MultiplexMode_Max', []),struct('Name', 'VCU_tireTempRRO','StartBit', [ 48;],'SignalSize', [ 16;],'ByteOrder', 'LittleEndian','ValueType', 'SIGNED','Class', 'int16','Signed', [ 1;],'Factor', [ 0.1;],'Offset', [ 0;],'Min', [ -3276.8;],'Max', [ 3276.7;],'Units', 'degC','StartVal', [ 0;],'Comment', 'RRO tire temperature','Multiplexed', [ 0;],'Multiplexor', [ 0;],'MultiplexMode_Min', [],'MultiplexMode_Max', [])}}  useSimFunc=0  sim_func_name=''  useStartVals=0
      settings: SourceProductName=Raptor
  raptor_function_call_collector : Raptor_lib/Triggers/raptor_function_call_collector  count=10
      settings: SourceProductName=Raptor
  wires:
  raptor_function_call_collector/1 -> RollingCounterGenerator/Trigger
  RollingCounterGenerator/1 -> raptor_can_txmsg/1
  Bus Selector/3 -> raptor_can_txmsg/4  "<IN_TireTempRRO_degC>"
  Bus Selector/2 -> raptor_can_txmsg/3  "<IN_TireTempRRM_degC>"
  Bus Selector/1 -> raptor_can_txmsg/2  "<IN_TireTempRRI_degC>"
  IO_CAN2_159_Bus/1 -> Bus Selector/1

== system IO/CANOutputs/Rear Rotor Temp ==
  IO_CAN2_155_Bus : Inport
  Bus Selector : BusSelector  OutputSignals=IN_RotorTempRL_degC,IN_RotorTempRR_degC
  RollingCounterGenerator : Utilities/RollingCounterGenerator
  raptor_can_txmsg : Raptor_lib/CAN/raptor_can_txmsg  canDefinition=struct('dbcFile', 'raptor_CAN2.dbc','message', 'VCU_155','comment', '','signals', {{'VCU_counterMsg155','VCU_rotorTempRL','VCU_rotorTempRR'}},'enabled', [ 1 1 1;],'scaled', [ 1 1 1;],'canBus', '''CAN2''','messageID', [ 155;],'idMask', [ 536870911;],'payloadMask', [],'payloadValue', [],'useDbcPeriod', [ 0;],'period', [ 100;],'queueSize', [ 1;],'label', [ 0;],'ver', [ 2;],'showID', [ 0;],'showRaw', [ 0;],'showRawMsg', [ 0;],'useStartVals', [ 0;],'extendedId', [ 0;],'useSimFunc', [ 0;],'sim_func_name', '''''','fill', [ 0;],'editID', [ 0;],'signalOrder', [ 1;],'signalAscDes', [ 1;],'msgLength', [ 8;])  canBus='CAN2'  queueSize=1  payloadMask=[]  payloadValue=[]  period=100  showID=0  label=0  idMask=hex2dec('1FFFFFFF')  fill=0  id=155  showRaw=0  signalOrder=1  signalInfo={{struct('Name', 'VCU_counterMsg155','StartBit', [ 0;],'SignalSize', [ 4;],'ByteOrder', 'LittleEndian','ValueType', 'UNSIGNED','Class', 'uint8','Signed', [ 0;],'Factor', [ 1;],'Offset', [ 0;],'Min', [ 0;],'Max', [ 15;],'Units', '','StartVal', [ 0;],'Comment', 'Counter Message 155','Multiplexed', [ 0;],'Multiplexor', [ 0;],'MultiplexMode_Min', [],'MultiplexMode_Max', []),struct('Name', 'VCU_rotorTempRL','StartBit', [ 16;],'SignalSize', [ 16;],'ByteOrder', 'LittleEndian','ValueType', 'SIGNED','Class', 'int16','Signed', [ 1;],'Factor', [ 0.1;],'Offset', [ 0;],'Min', [ -3276.8;],'Max', [ 3276.7;],'Units', 'degC','StartVal', [ 0;],'Comment', 'RL rotor temperature','Multiplexed', [ 0;],'Multiplexor', [ 0;],'MultiplexMode_Min', [],'MultiplexMode_Max', []),struct('Name', 'VCU_rotorTempRR','StartBit', [ 32;],'SignalSize', [ 16;],'ByteOrder', 'LittleEndian','ValueType', 'SIGNED','Class', 'int16','Signed', [ 1;],'Factor', [ 0.1;],'Offset', [ 0;],'Min', [ -3276.8;],'Max', [ 3276.7;],'Units', 'degC','StartVal', [ 0;],'Comment', 'RR rotor temperature','Multiplexed', [ 0;],'Multiplexor', [ 0;],'MultiplexMode_Min', [],'MultiplexMode_Max', [])}}  useSimFunc=0  sim_func_name=''  useStartVals=0
      settings: SourceProductName=Raptor
  raptor_function_call_collector : Raptor_lib/Triggers/raptor_function_call_collector  count=10
      settings: SourceProductName=Raptor
  wires:
  raptor_function_call_collector/1 -> RollingCounterGenerator/Trigger
  RollingCounterGenerator/1 -> raptor_can_txmsg/1
  Bus Selector/2 -> raptor_can_txmsg/3  "<IN_RotorTempRR_degC>"
  Bus Selector/1 -> raptor_can_txmsg/2  "<IN_RotorTempRL_degC>"
  IO_CAN2_155_Bus/1 -> Bus Selector/1

== system IO/CANOutputs/States ==
  IO_CAN2_152_Bus : Inport
  Bus Selector : BusSelector  OutputSignals=IO_DischargeContactorState_en,IO_MainMinusContactorState_en,IO_MainPlusContactorState_en,IO_PrechargeContactorState_en,IO_RTMSound_bool,IO_VehicleState_en
  RollingCounterGenerator : Utilities/RollingCounterGenerator
  raptor_can_txmsg : Raptor_lib/CAN/raptor_can_txmsg  canDefinition=struct('dbcFile', 'raptor_CAN2.dbc','message', 'VCU_152','comment', '','signals', {{'VCU_counterMsg152','VCU_dischargeContactorState','VCU_mainMinusContactorState','VCU_mainPlusContactorState','VCU_prechargeContactorState','VCU_rtmSound','VCU_vehicleState'}},'enabled', [ 1 1 1 1 1 1 1;],'scaled', [ 1 1 1 1 1 1 1;],'canBus', '''CAN2''','messageID', [ 152;],'idMask', [ 536870911;],'payloadMask', [],'payloadValue', [],'useDbcPeriod', [ 0;],'period', [ 100;],'queueSize', [ 1;],'label', [ 0;],'ver', [ 2;],'showID', [ 0;],'showRaw', [ 0;],'showRawMsg', [ 0;],'useStartVals', [ 0;],'extendedId', [ 0;],'useSimFunc', [ 0;],'sim_func_name', '''''','fill', [ 0;],'editID', [ 0;],'signalOrder', [ 1;],'signalAscDes', [ 1;],'msgLength', [ 8;])  canBus='CAN2'  queueSize=1  payloadMask=[]  payloadValue=[]  period=100  showID=0  label=0  idMask=hex2dec('1FFFFFFF')  fill=0  id=152  showRaw=0  signalOrder=1  signalInfo={{struct('Name', 'VCU_rtmSound','StartBit', [ 48;],'SignalSize', [ 1;],'ByteOrder', 'LittleEndian','ValueType', 'UNSIGNED','Class', 'uint8','Signed', [ 0;],'Factor', [ 1;],'Offset', [ 0;],'Min', [ 0;],'Max', [ 1;],'Units', '','StartVal', [ 0;],'Comment', 'Ready To Move sound','Multiplexed', [ 0;],'Multiplexor', [ 0;],'MultiplexMode_Min', [],'MultiplexMode_Max', []),struct('Name', 'VCU_mainMinusContactorState','StartBit', [ 40;],'SignalSize', [ 8;],'ByteOrder', 'LittleEndian','ValueType', 'UNSIGNED','Class', 'uint8','Signed', [ 0;],'Factor', [ 1;],'Offset', [ 0;],'Min', [ 0;],'Max', [ 255;],'Units', '','StartVal', [ 0;],'Comment', 'Main- contactor state','Multiplexed', [ 0;],'Multiplexor', [ 0;],'MultiplexMode_Min', [],'MultiplexMode_Max', []),struct('Name', 'VCU_mainPlusContactorState','StartBit', [ 32;],'SignalSize', [ 8;],'ByteOrder', 'LittleEndian','ValueType', 'UNSIGNED','Class', 'uint8','Signed', [ 0;],'Factor', [ 1;],'Offset', [ 0;],'Min', [ 0;],'Max', [ 255;],'Units', '','StartVal', [ 0;],'Comment', 'Main+ contactor state','Multiplexed', [ 0;],'Multiplexor', [ 0;],'MultiplexMode_Min', [],'MultiplexMode_Max', []),struct('Name', 'VCU_prechargeContactorState','StartBit', [ 24;],'SignalSize', [ 8;],'ByteOrder', 'LittleEndian','ValueType', 'UNSIGNED','Class', 'uint8','Signed', [ 0;],'Factor', [ 1;],'Offset', [ 0;],'Min', [ 0;],'Max', [ 255;],'Units', '','StartVal', [ 0;],'Comment', 'Precharge contactor state','Multiplexed', [ 0;],'Multiplexor', [ 0;],'MultiplexMode_Min', [],'MultiplexMode_Max', []),struct('Name', 'VCU_dischargeContactorState','StartBit', [ 16;],'SignalSize', [ 8;],'ByteOrder', 'LittleEndian','ValueType', 'UNSIGNED','Class', 'uint8','Signed', [ 0;],'Factor', [ 1;],'Offset', [ 0;],'Min', [ 0;],'Max', [ 255;],'Units', '','StartVal', [ 0;],'Comment', 'Discharge contactor state','Multiplexed', [ 0;],'Multiplexor', [ 0;],'MultiplexMode_Min', [],'MultiplexMode_Max', []),struct('Name', 'VCU_vehicleState','StartBit', [ 8;],'SignalSize', [ 8;],'ByteOrder', 'LittleEndian','ValueType', 'UNSIGNED','Class', 'uint8','Signed', [ 0;],'Factor', [ 1;],'Offset', [ 0;],'Min', [ 0;],'Max', [ 255;],'Units', '','StartVal', [ 0;],'Comment', 'Vehicle state','Multiplexed', [ 0;],'Multiplexor', [ 0;],'MultiplexMode_Min', [],'MultiplexMode_Max', []),struct('Name', 'VCU_counterMsg152','StartBit', [ 0;],'SignalSize', [ 4;],'ByteOrder', 'LittleEndian','ValueType', 'UNSIGNED','Class', 'uint8','Signed', [ 0;],'Factor', [ 1;],'Offset', [ 0;],'Min', [ 0;],'Max', [ 15;],'Units', '','StartVal', [ 0;],'Comment', 'Counter Message 152','Multiplexed', [ 0;],'Multiplexor', [ 0;],'MultiplexMode_Min', [],'MultiplexMode_Max', [])}}  useSimFunc=0  sim_func_name=''  useStartVals=0
      settings: SourceProductName=Raptor
  raptor_function_call_collector : Raptor_lib/Triggers/raptor_function_call_collector  count=10
      settings: SourceProductName=Raptor
  wires:
  Bus Selector/6 -> raptor_can_txmsg/7  "<IO_VehicleState_en>"
  Bus Selector/5 -> raptor_can_txmsg/6  "<IO_RTMSound_bool>"
  Bus Selector/4 -> raptor_can_txmsg/5  "<IO_PrechargeContactorState_en>"
  Bus Selector/3 -> raptor_can_txmsg/4  "<IO_MainPlusContactorState_en>"
  Bus Selector/2 -> raptor_can_txmsg/3  "<IO_MainMinusContactorState_en>"
  Bus Selector/1 -> raptor_can_txmsg/2  "<IO_DischargeContactorState_en>"
  raptor_function_call_collector/1 -> RollingCounterGenerator/Trigger
  RollingCounterGenerator/1 -> raptor_can_txmsg/1
  IO_CAN2_152_Bus/1 -> Bus Selector/1

== system IO/CANOutputs/Switches ==
  IO_CAN2_153_Bus : Inport
  Bus Selector : BusSelector  OutputSignals=IO_CoolSwitch_bool,IO_PwrDownSwitch_bool,IO_PwrUpSwitch_bool,IO_StartSwitch_bool
  RollingCounterGenerator : Utilities/RollingCounterGenerator
  raptor_can_txmsg : Raptor_lib/CAN/raptor_can_txmsg  canDefinition=struct('dbcFile', 'raptor_CAN2.dbc','message', 'VCU_153','comment', '','signals', {{'VCU_coolSwitch','VCU_counterMsg153','VCU_pwrDownSwitch','VCU_pwrUpSwitch','VCU_startSwitch'}},'enabled', [ 1 1 1 1 1;],'scaled', [ 1 1 1 1 1;],'canBus', '''CAN2''','messageID', [ 153;],'idMask', [ 536870911;],'payloadMask', [],'payloadValue', [],'useDbcPeriod', [ 0;],'period', [ 100;],'queueSize', [ 1;],'label', [ 0;],'ver', [ 2;],'showID', [ 0;],'showRaw', [ 0;],'showRawMsg', [ 0;],'useStartVals', [ 0;],'extendedId', [ 0;],'useSimFunc', [ 0;],'sim_func_name', '''''','fill', [ 0;],'editID', [ 0;],'signalOrder', [ 1;],'signalAscDes', [ 1;],'msgLength', [ 8;])  canBus='CAN2'  queueSize=1  payloadMask=[]  payloadValue=[]  period=100  showID=0  label=0  idMask=hex2dec('1FFFFFFF')  fill=0  id=153  showRaw=0  signalOrder=1  signalInfo={{struct('Name', 'VCU_coolSwitch','StartBit', [ 32;],'SignalSize', [ 1;],'ByteOrder', 'LittleEndian','ValueType', 'UNSIGNED','Class', 'uint8','Signed', [ 0;],'Factor', [ 1;],'Offset', [ 0;],'Min', [ 0;],'Max', [ 1;],'Units', '','StartVal', [ 0;],'Comment', 'Cool switch signal','Multiplexed', [ 0;],'Multiplexor', [ 0;],'MultiplexMode_Min', [],'MultiplexMode_Max', []),struct('Name', 'VCU_pwrDownSwitch','StartBit', [ 24;],'SignalSize', [ 1;],'ByteOrder', 'LittleEndian','ValueType', 'UNSIGNED','Class', 'uint8','Signed', [ 0;],'Factor', [ 1;],'Offset', [ 0;],'Min', [ 0;],'Max', [ 1;],'Units', '','StartVal', [ 0;],'Comment', 'Power down switch signal','Multiplexed', [ 0;],'Multiplexor', [ 0;],'MultiplexMode_Min', [],'MultiplexMode_Max', []),struct('Name', 'VCU_pwrUpSwitch','StartBit', [ 16;],'SignalSize', [ 1;],'ByteOrder', 'LittleEndian','ValueType', 'UNSIGNED','Class', 'uint8','Signed', [ 0;],'Factor', [ 1;],'Offset', [ 0;],'Min', [ 0;],'Max', [ 1;],'Units', '','StartVal', [ 0;],'Comment', 'Power up switch signal','Multiplexed', [ 0;],'Multiplexor', [ 0;],'MultiplexMode_Min', [],'MultiplexMode_Max', []),struct('Name', 'VCU_startSwitch','StartBit', [ 8;],'SignalSize', [ 1;],'ByteOrder', 'LittleEndian','ValueType', 'UNSIGNED','Class', 'uint8','Signed', [ 0;],'Factor', [ 1;],'Offset', [ 0;],'Min', [ 0;],'Max', [ 1;],'Units', '','StartVal', [ 0;],'Comment', 'Start switch signal','Multiplexed', [ 0;],'Multiplexor', [ 0;],'MultiplexMode_Min', [],'MultiplexMode_Max', []),struct('Name', 'VCU_counterMsg153','StartBit', [ 0;],'SignalSize', [ 4;],'ByteOrder', 'LittleEndian','ValueType', 'UNSIGNED','Class', 'uint8','Signed', [ 0;],'Factor', [ 1;],'Offset', [ 0;],'Min', [ 0;],'Max', [ 15;],'Units', '','StartVal', [ 0;],'Comment', 'Counter Message 153','Multiplexed', [ 0;],'Multiplexor', [ 0;],'MultiplexMode_Min', [],'MultiplexMode_Max', [])}}  useSimFunc=0  sim_func_name=''  useStartVals=0
      settings: SourceProductName=Raptor
  raptor_function_call_collector : Raptor_lib/Triggers/raptor_function_call_collector  count=10
      settings: SourceProductName=Raptor
  wires:
  raptor_function_call_collector/1 -> RollingCounterGenerator/Trigger
  RollingCounterGenerator/1 -> raptor_can_txmsg/2
  Bus Selector/4 -> raptor_can_txmsg/5  "<IO_StartSwitch_bool>"
  Bus Selector/3 -> raptor_can_txmsg/4  "<IO_PwrUpSwitch_bool>"
  Bus Selector/2 -> raptor_can_txmsg/3  "<IO_PwrDownSwitch_bool>"
  Bus Selector/1 -> raptor_can_txmsg/1  "<IO_CoolSwitch_bool>"
  IO_CAN2_153_Bus/1 -> Bus Selector/1

== system IO/CANOutputs/Throttle ==
  IO_CAN2_150_Bus : Inport
  Bus Selector : BusSelector  OutputSignals=IO_ThrottlePosition_pct,IO_ThrottlePosition1_pct,IO_ThrottlePosition2_pct
  RollingCounterGenerator : Utilities/RollingCounterGenerator
  raptor_can_txmsg : Raptor_lib/CAN/raptor_can_txmsg  canDefinition=struct('dbcFile', 'raptor_CAN2.dbc','message', 'VCU_150','comment', '','signals', {{'VCU_counterMsg150','VCU_throttlePosition','VCU_throttlePosition1','VCU_throttlePosition2'}},'enabled', [ 1 1 1 1;],'scaled', [ 1 1 1 1;],'canBus', '''CAN2''','messageID', [ 150;],'idMask', [ 536870911;],'payloadMask', [],'payloadValue', [],'useDbcPeriod', [ 0;],'period', [ 100;],'queueSize', [ 1;],'label', [ 0;],'ver', [ 2;],'showID', [ 0;],'showRaw', [ 0;],'showRawMsg', [ 0;],'useStartVals', [ 0;],'extendedId', [ 0;],'useSimFunc', [ 0;],'sim_func_name', '''''','fill', [ 0;],'editID', [ 0;],'signalOrder', [ 1;],'signalAscDes', [ 1;],'msgLength', [ 8;])  canBus='CAN2'  queueSize=1  payloadMask=[]  payloadValue=[]  period=100  showID=0  label=0  idMask=hex2dec('1FFFFFFF')  fill=0  id=150  showRaw=0  signalOrder=1  signalInfo={{struct('Name', 'VCU_throttlePosition2','StartBit', [ 48;],'SignalSize', [ 16;],'ByteOrder', 'LittleEndian','ValueType', 'SIGNED','Class', 'int16','Signed', [ 1;],'Factor', [ 0.1;],'Offset', [ 0;],'Min', [ 0;],'Max', [ 100;],'Units', '%','StartVal', [ 0;],'Comment', 'TPS2','Multiplexed', [ 0;],'Multiplexor', [ 0;],'MultiplexMode_Min', [],'MultiplexMode_Max', []),struct('Name', 'VCU_throttlePosition1','StartBit', [ 32;],'SignalSize', [ 16;],'ByteOrder', 'LittleEndian','ValueType', 'SIGNED','Class', 'int16','Signed', [ 1;],'Factor', [ 0.1;],'Offset', [ 0;],'Min', [ 0;],'Max', [ 100;],'Units', '%','StartVal', [ 0;],'Comment', 'TPS1','Multiplexed', [ 0;],'Multiplexor', [ 0;],'MultiplexMode_Min', [],'MultiplexMode_Max', []),struct('Name', 'VCU_throttlePosition','StartBit', [ 16;],'SignalSize', [ 16;],'ByteOrder', 'LittleEndian','ValueType', 'SIGNED','Class', 'int16','Signed', [ 1;],'Factor', [ 0.1;],'Offset', [ 0;],'Min', [ 0;],'Max', [ 100;],'Units', '%','StartVal', [ 0;],'Comment', 'Final throttle position','Multiplexed', [ 0;],'Multiplexor', [ 0;],'MultiplexMode_Min', [],'MultiplexMode_Max', []),struct('Name', 'VCU_counterMsg150','StartBit', [ 0;],'SignalSize', [ 4;],'ByteOrder', 'LittleEndian','ValueType', 'UNSIGNED','Class', 'uint8','Signed', [ 0;],'Factor', [ 1;],'Offset', [ 0;],'Min', [ 0;],'Max', [ 15;],'Units', '','StartVal', [ 0;],'Comment', 'Counter Message 150','Multiplexed', [ 0;],'Multiplexor', [ 0;],'MultiplexMode_Min', [],'MultiplexMode_Max', [])}}  useSimFunc=0  sim_func_name=''  useStartVals=0
      settings: SourceProductName=Raptor
  raptor_function_call_collector : Raptor_lib/Triggers/raptor_function_call_collector  count=10
      settings: SourceProductName=Raptor
  wires:
  raptor_function_call_collector/1 -> RollingCounterGenerator/Trigger
  RollingCounterGenerator/1 -> raptor_can_txmsg/1
  Bus Selector/3 -> raptor_can_txmsg/4  "<IO_ThrottlePosition2_pct>"
  Bus Selector/2 -> raptor_can_txmsg/3  "<IO_ThrottlePosition1_pct>"
  Bus Selector/1 -> raptor_can_txmsg/2  "<IO_ThrottlePosition_pct>"
  IO_CAN2_150_Bus/1 -> Bus Selector/1
